simulink model "FIR_InterpolationStream_Ex4"  (R2025a)
settings: Solver=VariableStepAuto  StartTime=0.0  StopTime=1  RelTol=1e-3
InitFcn:
  | SSR = 2;
  | Fs = 50e3;               % Sampling Frequency
  | Fpass = 16000;            % Passband Frequency
  | Fstop = 23000;            % Stopband Frequency
  | Dpass = 0.00460513763;    % Passband Ripple
  | Dstop = 0.0001;           % Stopband Attenuation
  | dens  = 16;                   % Density Factor
  | % Calculate the order from the parameters using FIRPMORD.
  | [N, Fo, Ao, W] = firpmord([Fpass, Fstop]/(Fs/2), [1 0], [Dpass, Dstop]);
  | % Calculate the coefficients using the FIRPM function.
  | b  = firpm(N, Fo, Ao, W, {dens});
  | coeffs = b;
undefined symbols (not defined in the file): None, S, vsva2197, xcvc1902
libraries: aieUtilities x4, dspsrcs4 x1, aieDSP x1, dspmlti4 x1, vmcUtilities x1
settings Model: Creator=sdegala  LastModifiedBy=sdegala
settings ModelReferenceCC: EnableRefExpFcnMdlSchedulingChecks=on
settings RTWCC: GPUComputeCapability=3.5

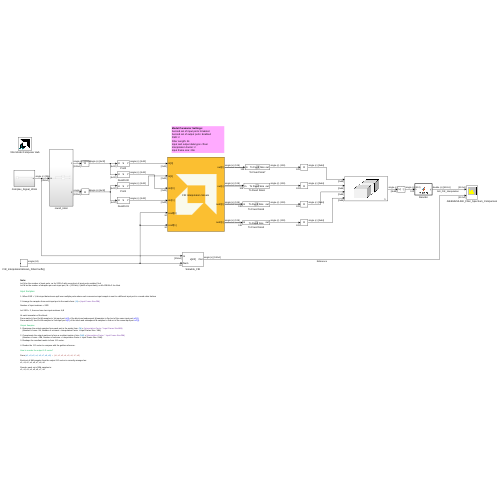
[thumbnail: Simulink's stored preview of the top-level diagram]
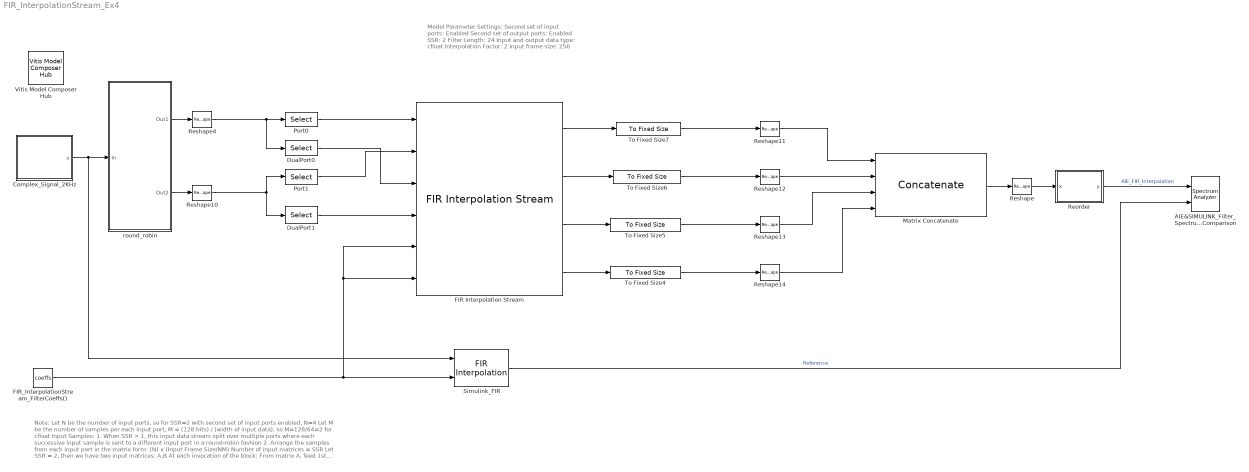
== system FIR_InterpolationStream_Ex4 ==
  note: Note:
      | Let N be the number of input ports, so for SSR=2 with second set of input ports enabled, N=4
      | Let M be the number of samples per each input port, M = (128 bits) / (width of input data), so M=128/64=2 for cfloat
      |
      | Input Samples:
      |
      | 1. When SSR > 1, this input data stream split over multiple ports where each successive input sample is sent to a different input port in a round-robin fashion
      |
      | 2. Arrange the samples from each input port in the matrix form: (N) x (Input Frame Size/NM)
      |
      | Number of input matrices = SSR
      |
      | Let SSR = 2, then we have two input matrices: A,B
      |
      | At each invocation of the block:
      | From matrix A, feed 1st M-samples to 1st input port in[0] of the block and subsequent M-samples to 2nd set of the same input port in2[0] .
      | From matrix B, feed 1st M-samples to 2nd input port in[1] of the block and subsequent M-samples to 2nd set of the same input port in2[1] .
      |
      | Output Samples:
      | 1. Rearrange the output samples from each port in the matrix form: (M) x (Interpolation Factor * Input Frame Size/NM)
      | (Number of rows = M, Number of columns = Interpolation Factor × Input Frame Size / NM).
      |
      | 2. Concatenate the output matrices to form a resultant matrix of size (NM) x (Interpolation Factor * Input Frame Size/NM)
      | (Number of rows = NM, Number of columns = Interpolation Factor × Input Frame Size / NM).
      | 3. Reshape the resultant matrix to form 1-D vector.
      |
      | 4. Reoder the 1-D vector to compare with the golden reference.
      |
      | How to reorder the output 1-D vector?
      |
      | From (x1, x3, x2, x4, x5, x7, x6, x8) → (x1, x2, x3, x4, x5, x6, x7, x8)
      |
      | Each set of NM samples from the output 1-D vector is currently arranged as:
      | x1, x3, x2, x4, x5, x7, x6, x8
      |
      | Reorder each set of NM samples to:
      | x1, x2, x3, x4, x5, x6, x7, x8.
  note: Model Parameter Settings:
      | Second set of input ports: Enabled
      | Second set of output ports: Enabled
      | SSR: 2
      | Filter Length: 24
      | Input and output data type: cfloat
      | Interpolation Factor: 2
      | Input frame size: 256
  AIE&SIMULINK_Filter_Spectrum_Comparison : SpectrumAnalyzer  NumInputPorts=2  WindowPosition=[490.000000,286.000000,800.000000,500.000000,]  Visible=on  ScopeFrameLocation=window  Span=49999.99999999999  StartFrequency=-24999.999999999996  StopFrequency=24999.999999999996  AveragingMethod=Exponential  YLimits=[-85.1987 36.07]  ShowLegend=on  ChannelNames="[\"\"]"  AllowFFTLengthLessThanSamplesPerUpdate=on  DefaultConfigurationName=spbscopes.SpectrumAnalyzerBlockCfg
  Complex_Signal_2KHz : Subsystem
  DualPort0 : Selector  NumberOfDimensions=2  InputPortWidth=256/SSR  IndexOptions=Index vector (dialog),Select all  Indices=[3 4],1  OutputSizes=1,1
  DualPort1 : Selector  NumberOfDimensions=2  InputPortWidth=256/SSR  IndexOptions=Index vector (dialog),Select all  Indices=[3 4],1  OutputSizes=1,1
  FIR Interpolation Stream : aieDSP/FIR Interpolation Stream  data_type=cfloat  coef_type=float  use_coeff_reload=on  dual_ip=on  num_outputs=on  coeff=coeffs  fir_length=24  interpolate_factor=2  input_window_size=256  shift_val=0  rnd_mode=Round to positive infinity  sat_mode=0-None  ssr=SSR  interp_poly=1  casc_length=1  AIE_VARIANT=1  TP_API=1  blockJsonConstraints=[]  blockJsonConstraintsInternal=[]  spec=vmc_stream_fir_interpolate_asym.json  SerializedMaskParamNames=[]  SerializedMaskParamValues=[]  SerializedMaskParamVisibilities=[]  block_type=FIR Interpolation Stream  SerializedMaskParamDataypes=typename|typename|uint|uint|uint|coef_type|uint|uint|uint|uint|uint|uint|uint|uint|uint|uint|uint  SerializedMaskParamEnumStrArr=0|0|0|0|0|0|0|0|0|0|Floor,Ceiling,Round to positive infinity,Round to negative infinity,Round symmetrical to infinity,Round symmetrical to zero,Round convergent to even,Round convergent to odd|0-None,1-Asymmetric,3-Symmetric|0|0|0|0|0  SerializedMaskParamEnumValArr=0|0|0|0|0|0|0|0|0|0|0,1,2,3,4,5,6,7|0,1,3|0|0|0|0|0  SerializedMaskParamVectorArr=0|0|0|0|0|1|0|0|0|0|0|0|0|0|0|0|0  SerializedMaskParamKeys=TT_DATA|TT_COEFF|TP_USE_COEFF_RELOAD|TP_DUAL_IP|TP_NUM_OUTPUTS|coeff|TP_FIR_LEN|TP_INTERPOLATE_FACTOR|TP_INPUT_WINDOW_VSIZE|TP_SHIFT|TP_RND|TP_SAT|TP_SSR|TP_PARA_INTERP_POLY|TP_CASC_LEN|AIE_VARIANT|TP_API
  FIR_InterpolationStream_FilterCoeffs() : Constant  Value=coeffs  OutDataTypeStr=single
  Matrix Concatenate : Concatenate  NumInputs=4  Mode=Multidimensional array
  Port0 : Selector  NumberOfDimensions=2  InputPortWidth=(256/SSR)  IndexOptions=Index vector (dialog),Select all  Indices=[1 2],1  OutputSizes=1,1
  Port1 : Selector  NumberOfDimensions=2  InputPortWidth=(256/SSR)  IndexOptions=Index vector (dialog),Select all  Indices=[1 2],1  OutputSizes=1,1
  Reorder : MATLAB Function  TreatAsAtomicUnit=on
  Reshape : Reshape
  Reshape10 : Reshape  OutputDimensionality=Customize  OutputDimensions=[4,32]
  Reshape{11..14} (4 alike) : Reshape  OutputDimensionality=Customize  OutputDimensions=[2,64]
  Reshape4 : Reshape  OutputDimensionality=Customize  OutputDimensions=[4,32]
  "Simulink_FIR " : dspmlti4/FIR Interpolation  FilterSource=Input port  PrivateCoeffs=0  h=coeffs  L=2  FilterObject=FINTERP  InputProcessing=Columns as channels (frame based)  framing=Enforce single-rate processing  outputBufInitCond=0  roundingMode=Ceiling  overflowMode=off  firstCoeffDataTypeStr=Inherit: Same word length as input  firstCoeffMin=[]  firstCoeffMax=[]  firstCoeffLastDataTypeStr=Inherit: Same word length as input  outputMin=[]  outputMax=[]
  To Fixed Size{4..7} (4 alike) : aieUtilities/To Fixed Size  Mode=Stop simulation when input variable-size signal is not full  OutputSize=Inherit: Same as input  CopyMethod=Buffer samples to form output  HasStatusOutput=on
  Vitis Model Composer Hub : vmcUtilities/Vitis Model Composer Hub  Tag=genX  CodeGeneration=off  StartColumn=1  NumberOfColumns=1  TargetDirectory=./code  exportDesign=off  analyzeDesign=off  validateDesignOnHw=off  ExportType=AI Engines  IpVendor=xilinx.com  IpLibrary=hls  IpVersion=1.0  IpHWLanguage=Verilog  AieCompilerOptions={}  AieSimulatorOptions={}  CreateTestbench=off  TestbenchStackSize=10  RunRtlSim=off  RunCSim=off  RunAieSim=off  AieSimTimeout=50000  RunAieSimProfiling=off  LaunchVitisAnalyzer=off  PlotOutput=off  RunX86Sim=off  X86SimTimeout=10  GenHwImage=off  GenLibadfXo=off  GenHwValidationCode=off  PlatformType=Not Specified  HwSystemType=Baremetal  HwValidationTarget=hw  ProjDevice=xcvc1902-vsva2197-1LP-e-S  ProjDevicePart=xcvc1902-vsva2197-1LP-e-S  AIEType=AIE  SamplePeriod=-1  ClockFrequency=200  DataPathParallelism=1  xilinxfamily=versalaicore  part=xcvc1902  speed=-1LP-e-S  package=vsva2197  directory=./netlist  testbench=off  incr_netlist=off  synthesis_tool=Vivado  clock_wrapper=Clock Enables  dbl_ovrd=According to Block Masks  dcm_input_clock_period=10  sysclk_period=10  simulink_period=1  eval_field=0  LogFileName=''  NThreads=4
  round_robin : Subsystem
  wires:
  FIR_InterpolationStream_FilterCoeffs()/1 -> FIR Interpolation Stream/5, FIR Interpolation Stream/6, "Simulink_FIR "/2
  round_robin/1(Out1) -> Reshape4/1
  round_robin/2(Out2) -> Reshape10/1
  Port0/1 -> FIR Interpolation Stream/1
  Port1/1 -> FIR Interpolation Stream/2
  DualPort0/1 -> FIR Interpolation Stream/3
  DualPort1/1 -> FIR Interpolation Stream/4
  Complex_Signal_2KHz/1(u) -> "Simulink_FIR "/1, round_robin/1(in)
  Reshape4/1 -> DualPort0/1, Port0/1
  Reshape10/1 -> DualPort1/1, Port1/1
  "Simulink_FIR "/1 -> AIE&SIMULINK_Filter_Spectrum_Comparison/2  "Reference"
  Reshape11/1 -> Matrix Concatenate/1
  To Fixed Size7/1 -> Reshape11/1
  To Fixed Size5/1 -> Reshape13/1
  To Fixed Size6/1 -> Reshape12/1
  To Fixed Size4/1 -> Reshape14/1
  FIR Interpolation Stream/1 -> To Fixed Size7/1
  FIR Interpolation Stream/2 -> To Fixed Size6/1
  FIR Interpolation Stream/3 -> To Fixed Size5/1
  FIR Interpolation Stream/4 -> To Fixed Size4/1
  Reorder/1(y) -> AIE&SIMULINK_Filter_Spectrum_Comparison/1  "AIE_FIR_Interpolation"
  Matrix Concatenate/1 -> Reshape/1
  Reshape12/1 -> Matrix Concatenate/2
  Reshape13/1 -> Matrix Concatenate/3
  Reshape14/1 -> Matrix Concatenate/4
  Reshape/1 -> Reorder/1(x)

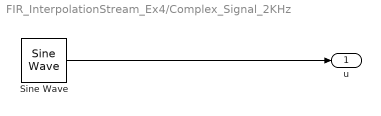
== system FIR_InterpolationStream_Ex4/Complex_Signal_2KHz ==
  Sine Wave : dspsrcs4/Sine Wave  Amplitude=1  Frequency=2e3  Phase=0  SampleMode=Discrete  OutComplex=Complex  CompMethod=Trigonometric fcn  TableSize=Speed  SampleTime=1/25e3  SamplesPerFrame=256  ResetState=Restart at time zero  OutputFrames=off  dataType=single  wordLen=16  udDataType=sfix(16)  fracBitsMode=Best precision  numFracBits=15  OutDataTypeStr=single  LastOutDataTypeStr=single
  u : Outport
  wires:
  Sine Wave/1 -> u/1

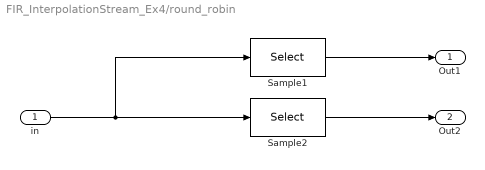
== system FIR_InterpolationStream_Ex4/round_robin ==
  in : Inport
  Sample1 : Selector  InputPortWidth=256  IndexOptions=Index vector (dialog)  Indices=1:SSR:256  OutputSizes=1
  Sample2 : Selector  InputPortWidth=256  IndexOptions=Index vector (dialog)  Indices=2:SSR:256  OutputSizes=1
  Out1 : Outport
  Out2 : Outport  Port=2
  wires:
  in/1 -> Sample2/1, Sample1/1
  Sample2/1 -> Out2/1
  Sample1/1 -> Out1/1

== matlab function FIR_InterpolationStream_Ex4/Reorder ==
  data: x input; y output
function y = reorder(x)
y = complex(zeros(512,1));
   count = 0;
for i = 1:8:512
 
y(i:i+7,1) = x([count+1 count+3 count+2 count+4 count+5 count+7 count+6 count+8]);
count = count + 8;
end
